simulink model "mech_robot_vr"  (Simulink 7.1)
settings: Solver=ode15s  StartTime=0.0  StopTime=1  RelTol=1e-3  AbsTol=1e-4
PreLoadFcn:
  | load mech_robot_images;mech_robot_data;
undefined symbols (not defined in the file or in its folder): Actuator, rad, s
libraries: mblibv1 x88
(part 3 of 4)

== system mech_robot_vr/Robot/Link 2/Drive2/Continuous angle ==
  Continuous Angle : Subsystem  Tag=Factory continuousAngle  Orientation=left  AncestorBlock=mblibv1/Utilities/Continuous Angle  mask{rad=rad, rads=rad/s}
      mask prompts: rad "Angle measured in:"; rads "Rate measured in:"
      mask help: Outputs a continuous, unbounded angle given a discontinuous, bounded angle and the angular velocity. Choose units for the angle and the angular velocity (rate).
      mask Help: web(mech_help('continuousangle'))
      mask StyleString: popup(rad|deg),popup(rad/s|deg/s)
  Demux : Demux  Orientation=left  Outputs=2
  Joint Sensor : mblibv1/Sensors &  Actuators/Joint Sensor  Orientation=left  DialogController=MECH.DynMechDlgSource  SystemSampleTime=-1  PhysicalDomain=Mechanical  PortType=blob  Muxed=on  Pose=off  Angle=on  AngleUnits=rad  ArcVelocity=on  ArcVelocityUnits=rad/s  ArcAcceleration=off  ArcAccelerationUnits=deg/s^2  CoordPosition=on  CoordPositionUnits=m  Velocity=off  VelocityUnits=m/s  Acceleration=off  AccelerationUnits=m/s^2  Quaternion=on  QuaternionDT=off  QuaternionDDT=off  QuaternionUnits=off  OutputVector=[ 1 1 ]  ActiveIO=on  Width=2  DialogClass=MechanicalSensorBlock  Primitive=R1  Force=off  ForceUnits=N  Torque=off  TorqueUnits=N-m  ReferenceFrame=Absolute (INERTIAL)  ReactionSensedSide=Base  ReactionReferenceFrame=Absolute (World)  ReactionForce=off  ReactionForceUnits=N  ReactionMoment=off  ReactionMomentUnits=N-m
  Mux : Mux  Orientation=left  Inputs=2
  In : PMIOPort  Orientation=left  Port=1  Side=Left
  Out : Outport  Orientation=left  OutDataType=sfix(16)  OutScaling=2^0
  phi : Outport  Orientation=left  Port=2  OutDataType=sfix(16)  OutScaling=2^0
  wires:
  Mux/1 -> Out/1
  Continuous Angle/1(Continuous Angle) -> Mux/1, phi/1
  Demux/2 -> Mux/2, Continuous Angle/2(Rate)
  Demux/1 -> Continuous Angle/1(Angle)
  Joint Sensor/1 -> Demux/1
  connections:
  In/RConn1 -- Joint Sensor/LConn1

== system mech_robot_vr/Robot/Link 2/Drive2/Continuous angle  ==
  Continuous Angle : mblibv1/Utilities/Continuous Angle  Tag=Factory continuousAngle  Orientation=left  SystemSampleTime=-1  rad=rad  rads=rad/s
  Demux : Demux  Orientation=left  Outputs=2
  Gain2 : Gain  Orientation=left  Gain=Actuator.GearRatio  ParameterDataType=sfix(16)  ParameterScaling=2^0  OutDataType=sfix(16)  OutScaling=2^0  SaturateOnIntegerOverflow=on  OutDataTypeStr=Inherit: Same as input  ParamDataTypeStr=Inherit: Same as input
  Joint Sensor : mblibv1/Sensors &  Actuators/Joint Sensor  Orientation=left  DialogController=MECH.DynMechDlgSource  SystemSampleTime=-1  PhysicalDomain=Mechanical  PortType=blob  Muxed=on  Pose=off  Angle=on  AngleUnits=rad  ArcVelocity=on  ArcVelocityUnits=rad/s  ArcAcceleration=off  ArcAccelerationUnits=deg/s^2  CoordPosition=on  CoordPositionUnits=m  Velocity=off  VelocityUnits=m/s  Acceleration=off  AccelerationUnits=m/s^2  Quaternion=on  QuaternionDT=off  QuaternionDDT=off  QuaternionUnits=off  OutputVector=[ 1 1 ]  ActiveIO=on  Width=2  DialogClass=MechanicalSensorBlock  Primitive=R1  Force=off  ForceUnits=N  Torque=off  TorqueUnits=N-m  ReferenceFrame=Absolute (INERTIAL)  ReactionSensedSide=Base  ReactionReferenceFrame=Absolute (World)  ReactionForce=off  ReactionForceUnits=N  ReactionMoment=off  ReactionMomentUnits=N-m
  Mux : Mux  Orientation=left  Inputs=2
  To Workspace : ToWorkspace  VariableName=Body2_D  SampleTime=-1  SaveFormat=Structure With Time
  In : PMIOPort  Orientation=left  Port=1  Side=Left
  "Out " : Outport  Orientation=left  OutDataType=sfix(16)  OutScaling=2^0
  tag scope: Body2=global
  wires:
  Joint Sensor/1 -> Demux/1
  Demux/1 -> Continuous Angle/1
  Demux/2 -> Continuous Angle/2, Mux/2
  Continuous Angle/1 -> Mux/1, [Body2], To Workspace/1
  Mux/1 -> Gain2/1
  Gain2/1 -> "Out "/1
  connections:
  In/RConn1 -- Joint Sensor/LConn1

== system mech_robot_vr/Robot/Link 2/Drive2/Controller ==
  Angular velocity : Inport  OutDataType=sfix(16)  OutScaling=2^0
  w_ref : Inport  Orientation=down  Port=2  OutDataType=sfix(16)  OutScaling=2^0
  phi_ref : Inport  Port=3  OutDataType=sfix(16)  OutScaling=2^0
  phi : Inport  Port=4  OutDataType=sfix(16)  OutScaling=2^0
  Integrator : Integrator  ZeroCross=off
  Lead filter : TransferFcn  Numerator=[340.8*9.95e-3 340.8]  Denominator=[0.56e-3 1]
  Position gain : Gain  Gain=0.3  ParameterDataType=sfix(16)  ParameterScaling=2^0  OutDataType=sfix(16)  OutScaling=2^0  SaturateOnIntegerOverflow=on  OutDataTypeStr=Inherit: Same as input  ParamDataTypeStr=Inherit: Same as input
  Rate controller : TransferFcn  Orientation=up  Numerator=[40e-3 1]  Denominator=[20.2e-3 1]
  Sum : Sum  Inputs=|+-  OutDataType=sfix(16)  OutScaling=2^0  SaturateOnIntegerOverflow=on
  Sum1 : Sum  Inputs=++|  OutDataType=sfix(16)  OutScaling=2^0  SaturateOnIntegerOverflow=on
  Sum2 : Sum  Inputs=|+-  OutDataType=sfix(16)  OutScaling=2^0  SaturateOnIntegerOverflow=on
  Tacho filter : TransferFcn  Numerator=0.03  Denominator="[8.475e-4  1]"
  Taco dynamics : TransferFcn  Numerator=1  Denominator="[1/(2014*2014)   2*0.294/2014  1]"
  Velocity gain : Gain  Orientation=down  Gain=0.03  ParameterDataType=sfix(16)  ParameterScaling=2^0  OutDataType=sfix(16)  OutScaling=2^0  SaturateOnIntegerOverflow=on  OutDataTypeStr=Inherit: Same as input  ParamDataTypeStr=Inherit: Same as input
  i_ref : Outport  OutDataType=sfix(16)  OutScaling=2^0
  wires:
  phi_ref/1 -> Sum/1
  Sum/1 -> Position gain/1
  Position gain/1 -> Sum1/2
  Velocity gain/1 -> Sum1/1
  Sum1/1 -> Sum2/1
  Sum2/1 -> Lead filter/1
  Rate controller/1 -> Sum2/2
  Taco dynamics/1 -> Rate controller/1
  Tacho filter/1 -> Taco dynamics/1
  Angular velocity/1 -> Tacho filter/1
  Lead filter/1 -> Integrator/1
  Integrator/1 -> i_ref/1
  w_ref/1 -> Velocity gain/1
  phi/1 -> Sum/2

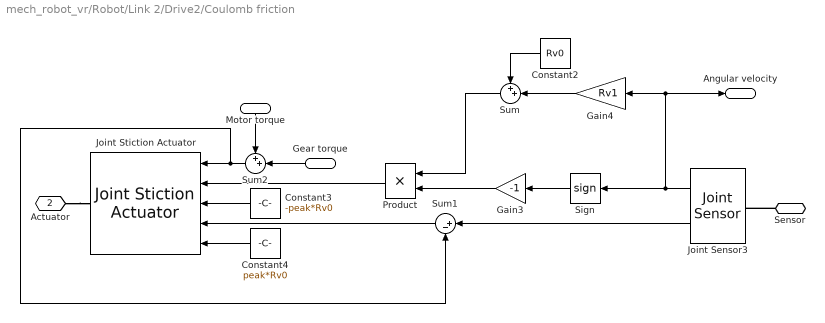
== system mech_robot_vr/Robot/Link 2/Drive2/Coulomb friction ==
  Motor torque : Inport  Orientation=down  OutDataType=sfix(16)  OutScaling=2^0
  Gear torque : Inport  Orientation=left  Port=2  OutDataType=sfix(16)  OutScaling=2^0
  Constant2 : Constant  Orientation=left  Value=Rv0  OutDataType=sfix(16)  OutScaling=2^0
  Constant3 : Constant  Orientation=left  Value=-peak*Rv0  OutDataType=sfix(16)  OutScaling=2^0
  Constant4 : Constant  Orientation=left  Value=peak*Rv0  OutDataType=sfix(16)  OutScaling=2^0
  Gain3 : Gain  Orientation=left  Gain=-1  ParameterDataType=sfix(16)  ParameterScaling=2^0  OutDataType=sfix(16)  OutScaling=2^0  SaturateOnIntegerOverflow=on  OutDataTypeStr=Inherit: Same as input  ParamDataTypeStr=Inherit: Same as input
  Gain4 : Gain  Orientation=left  Gain=Rv1  ParameterDataType=sfix(16)  ParameterScaling=2^0  OutDataType=sfix(16)  OutScaling=2^0  SaturateOnIntegerOverflow=on  OutDataTypeStr=Inherit: Same as input  ParamDataTypeStr=Inherit: Same as input
  Joint Sensor3 : mblibv1/Sensors &  Actuators/Joint Sensor  Description=Mechanical Blockset  Orientation=left  DialogController=MECH.DynMechDlgSource  SystemSampleTime=-1  PhysicalDomain=Mechanical  PortType=blob  Muxed=off  Pose=off  Angle=off  AngleUnits=rad  ArcVelocity=on  ArcVelocityUnits=rad/s  ArcAcceleration=off  ArcAccelerationUnits=deg/s^2  CoordPosition=off  CoordPositionUnits=m  Velocity=off  VelocityUnits=m/s  Acceleration=off  AccelerationUnits=m/s^2  Quaternion=off  QuaternionDT=off  QuaternionDDT=off  QuaternionUnits=off  OutputVector=[ 1 1 ]  ActiveIO=on  Width=2  DialogClass=MechanicalSensorBlock  Primitive=R1  Force=off  ForceUnits=N  Torque=on  TorqueUnits=N-m  ReferenceFrame=Absolute (INERTIAL)  ReactionSensedSide=Base  ReactionReferenceFrame=Absolute (World)  ReactionForce=off  ReactionForceUnits=N  ReactionMoment=off  ReactionMomentUnits=N-m
  Joint Stiction Actuator : mblibv1/Sensors &  Actuators/Joint Stiction Actuator  Description=Mechanical Blockset  Orientation=left  DialogController=MECH.DynMechDlgSource  SystemSampleTime=-1  PhysicalDomain=Mechanical  PortType=blob  ActuationStyle=Force  AngleUnits=deg  ArcVelocityUnits=deg/s  ArcAccelerationUnits=deg/s^2  CoordPositionUnits=m  VelocityUnits=m/s  AccelerationUnits=m/s^2  ForceUnits=N  TorqueUnits=N-m  ActiveIO=on  Width=5  DialogClass=EventActuatorBlock  Primitive=R1  FrictionalForceUnits=N  ExternalForceUnits=N  FrictionalTorqueUnits=N-m  ExternalTorqueUnits=N-m  LockingTolerance=1e-3
  Product : Product  Orientation=left  OutDataType=sfix(16)  OutScaling=2^0  SaturateOnIntegerOverflow=on  InputSameDT=on  OutDataTypeStr=Inherit: Same as first input
  Sign : Signum  Orientation=left
  Sum : Sum  Orientation=left  Inputs=++|  OutDataType=sfix(16)  OutScaling=2^0  SaturateOnIntegerOverflow=on  InputSameDT=on  OutDataTypeStr=Inherit: Same as first input
  Sum1 : Sum  Orientation=left  Inputs=|+-  OutDataType=sfix(16)  OutScaling=2^0  SaturateOnIntegerOverflow=on  InputSameDT=on  OutDataTypeStr=Inherit: Same as first input
  Sum2 : Sum  Orientation=left  Inputs=++|  OutDataType=sfix(16)  OutScaling=2^0  SaturateOnIntegerOverflow=on
  Sensor : PMIOPort  Orientation=left  Port=1  Side=Right
  Actuator : PMIOPort  Port=2  Side=Right
  Angular velocity : Outport  OutDataType=sfix(16)  OutScaling=2^0
  wires:
  Sum1/1 -> Joint Stiction Actuator/4
  Constant3/1 -> Joint Stiction Actuator/3
  Gain3/1 -> Product/2
  Constant2/1 -> Sum/1
  Gain4/1 -> Sum/2
  Constant4/1 -> Joint Stiction Actuator/5
  Joint Sensor3/2 -> Sum1/1
  Sum/1 -> Product/1
  Sign/1 -> Gain3/1
  Product/1 -> Joint Stiction Actuator/2
  Motor torque/1 -> Sum2/1
  Gear torque/1 -> Sum2/2
  Sum2/1 -> Joint Stiction Actuator/1, Sum1/2
  Joint Sensor3/1 -> Sign/1, Gain4/1, Angular velocity/1
  connections:
  Sensor/RConn1 -- Joint Sensor3/LConn1
  Actuator/RConn1 -- Joint Stiction Actuator/RConn1

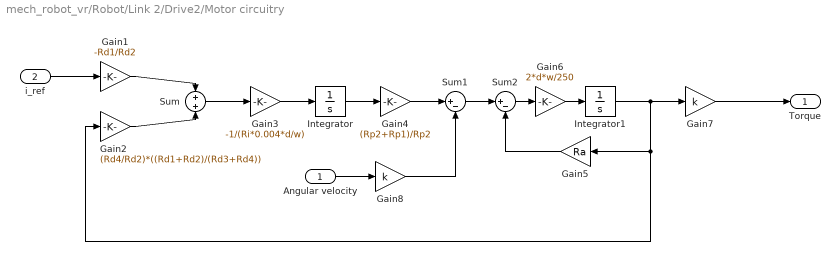
== system mech_robot_vr/Robot/Link 2/Drive2/Motor circuitry ==
  Angular velocity : Inport  OutDataType=sfix(16)  OutScaling=2^0
  i_ref : Inport  Port=2  OutDataType=sfix(16)  OutScaling=2^0
  Gain1 : Gain  Gain=-Rd1/Rd2  ParameterDataType=sfix(16)  ParameterScaling=2^0  OutDataType=sfix(16)  OutScaling=2^0  SaturateOnIntegerOverflow=on  OutDataTypeStr=Inherit: Same as input  ParamDataTypeStr=Inherit: Same as input
  Gain2 : Gain  Gain=(Rd4/Rd2)*((Rd1+Rd2)/(Rd3+Rd4))  ParameterDataType=sfix(16)  ParameterScaling=2^0  OutDataType=sfix(16)  OutScaling=2^0  SaturateOnIntegerOverflow=on  OutDataTypeStr=Inherit: Same as input  ParamDataTypeStr=Inherit: Same as input
  Gain3 : Gain  Gain=-1/(Ri*0.004*d/w)  ParameterDataType=sfix(16)  ParameterScaling=2^0  OutDataType=sfix(16)  OutScaling=2^0  SaturateOnIntegerOverflow=on  OutDataTypeStr=Inherit: Same as input  ParamDataTypeStr=Inherit: Same as input
  Gain4 : Gain  Gain=(Rp2+Rp1)/Rp2  ParameterDataType=sfix(16)  ParameterScaling=2^0  OutDataType=sfix(16)  OutScaling=2^0  SaturateOnIntegerOverflow=on  OutDataTypeStr=Inherit: Same as input  ParamDataTypeStr=Inherit: Same as input
  Gain5 : Gain  Orientation=left  Gain=Ra  ParameterDataType=sfix(16)  ParameterScaling=2^0  OutDataType=sfix(16)  OutScaling=2^0  SaturateOnIntegerOverflow=on  OutDataTypeStr=Inherit: Same as input  ParamDataTypeStr=Inherit: Same as input
  Gain6 : Gain  Gain=2*d*w/250  ParameterDataType=sfix(16)  ParameterScaling=2^0  OutDataType=sfix(16)  OutScaling=2^0  SaturateOnIntegerOverflow=on  OutDataTypeStr=Inherit: Same as input  ParamDataTypeStr=Inherit: Same as input
  Gain7 : Gain  Gain=k  ParameterDataType=sfix(16)  ParameterScaling=2^0  OutDataType=sfix(16)  OutScaling=2^0  SaturateOnIntegerOverflow=on  OutDataTypeStr=Inherit: Same as input  ParamDataTypeStr=Inherit: Same as input
  Gain8 : Gain  Gain=k  ParameterDataType=sfix(16)  ParameterScaling=2^0  OutDataType=sfix(16)  OutScaling=2^0  SaturateOnIntegerOverflow=on  OutDataTypeStr=Inherit: Same as input  ParamDataTypeStr=Inherit: Same as input
  Integrator : Integrator  ZeroCross=off
  Integrator1 : Integrator  ZeroCross=off
  Sum : Sum  OutDataType=sfix(16)  OutScaling=2^0  SaturateOnIntegerOverflow=on  InputSameDT=on  OutDataTypeStr=Inherit: Same as first input
  Sum1 : Sum  Inputs=|+-  OutDataType=sfix(16)  OutScaling=2^0  SaturateOnIntegerOverflow=on  InputSameDT=on  OutDataTypeStr=Inherit: Same as first input
  Sum2 : Sum  Inputs=|+-  OutDataType=sfix(16)  OutScaling=2^0  SaturateOnIntegerOverflow=on  InputSameDT=on  OutDataTypeStr=Inherit: Same as first input
  Torque : Outport  OutDataType=sfix(16)  OutScaling=2^0
  wires:
  Angular velocity/1 -> Gain8/1
  Gain8/1 -> Sum1/2
  Gain6/1 -> Integrator1/1
  Sum2/1 -> Gain6/1
  Gain5/1 -> Sum2/2
  Integrator1/1 -> Gain2/1, Gain5/1, Gain7/1
  Sum1/1 -> Sum2/1
  Gain4/1 -> Sum1/1
  Integrator/1 -> Gain4/1
  Gain3/1 -> Integrator/1
  Sum/1 -> Gain3/1
  Gain2/1 -> Sum/2
  Gain1/1 -> Sum/1
  i_ref/1 -> Gain1/1
  Gain7/1 -> Torque/1

== system mech_robot_vr/Robot/Link3/Drive3/Continuous angle ==
  Continuous Angle : Subsystem  Tag=Factory continuousAngle  Orientation=left  AncestorBlock=mblibv1/Utilities/Continuous Angle  mask{rad=rad, rads=rad/s}
      mask prompts: rad "Angle measured in:"; rads "Rate measured in:"
      mask help: Outputs a continuous, unbounded angle given a discontinuous, bounded angle and the angular velocity. Choose units for the angle and the angular velocity (rate).
      mask Help: web(mech_help('continuousangle'))
      mask StyleString: popup(rad|deg),popup(rad/s|deg/s)
  Demux : Demux  Orientation=left  Outputs=2
  Joint Sensor : mblibv1/Sensors &  Actuators/Joint Sensor  Orientation=left  DialogController=MECH.DynMechDlgSource  SystemSampleTime=-1  PhysicalDomain=Mechanical  PortType=blob  Muxed=on  Pose=off  Angle=on  AngleUnits=rad  ArcVelocity=on  ArcVelocityUnits=rad/s  ArcAcceleration=off  ArcAccelerationUnits=deg/s^2  CoordPosition=on  CoordPositionUnits=m  Velocity=off  VelocityUnits=m/s  Acceleration=off  AccelerationUnits=m/s^2  Quaternion=on  QuaternionDT=off  QuaternionDDT=off  QuaternionUnits=off  OutputVector=[ 1 1 ]  ActiveIO=on  Width=2  DialogClass=MechanicalSensorBlock  Primitive=R1  Force=off  ForceUnits=N  Torque=off  TorqueUnits=N-m  ReferenceFrame=Absolute (INERTIAL)  ReactionSensedSide=Base  ReactionReferenceFrame=Absolute (World)  ReactionForce=off  ReactionForceUnits=N  ReactionMoment=off  ReactionMomentUnits=N-m
  Mux : Mux  Orientation=left  Inputs=2
  In : PMIOPort  Orientation=left  Port=1  Side=Left
  Out : Outport  Orientation=left  OutDataType=sfix(16)  OutScaling=2^0
  phi : Outport  Orientation=left  Port=2  OutDataType=sfix(16)  OutScaling=2^0
  wires:
  Mux/1 -> Out/1
  Continuous Angle/1(Continuous Angle) -> Mux/1, phi/1
  Demux/2 -> Mux/2, Continuous Angle/2(Rate)
  Demux/1 -> Continuous Angle/1(Angle)
  Joint Sensor/1 -> Demux/1
  connections:
  In/RConn1 -- Joint Sensor/LConn1

== system mech_robot_vr/Robot/Link3/Drive3/Continuous angle  ==
  Continuous Angle : mblibv1/Utilities/Continuous Angle  Tag=Factory continuousAngle  Orientation=left  SystemSampleTime=-1  rad=rad  rads=rad/s
  Demux : Demux  Orientation=left  Outputs=2
  Gain2 : Gain  Orientation=left  Gain=Actuator.GearRatio  ParameterDataType=sfix(16)  ParameterScaling=2^0  OutDataType=sfix(16)  OutScaling=2^0  SaturateOnIntegerOverflow=on  OutDataTypeStr=Inherit: Same as input  ParamDataTypeStr=Inherit: Same as input
  Joint Sensor : mblibv1/Sensors &  Actuators/Joint Sensor  Orientation=left  DialogController=MECH.DynMechDlgSource  SystemSampleTime=-1  PhysicalDomain=Mechanical  PortType=blob  Muxed=on  Pose=off  Angle=on  AngleUnits=rad  ArcVelocity=on  ArcVelocityUnits=rad/s  ArcAcceleration=off  ArcAccelerationUnits=deg/s^2  CoordPosition=on  CoordPositionUnits=m  Velocity=off  VelocityUnits=m/s  Acceleration=off  AccelerationUnits=m/s^2  Quaternion=on  QuaternionDT=off  QuaternionDDT=off  QuaternionUnits=off  OutputVector=[ 1 1 ]  ActiveIO=on  Width=2  DialogClass=MechanicalSensorBlock  Primitive=R1  Force=off  ForceUnits=N  Torque=off  TorqueUnits=N-m  ReferenceFrame=Absolute (INERTIAL)  ReactionSensedSide=Base  ReactionReferenceFrame=Absolute (World)  ReactionForce=off  ReactionForceUnits=N  ReactionMoment=off  ReactionMomentUnits=N-m
  Mux : Mux  Orientation=left  Inputs=2
  To Workspace : ToWorkspace  VariableName=Body3_D  SampleTime=-1  SaveFormat=Structure With Time
  In : PMIOPort  Orientation=left  Port=1  Side=Left
  "Out " : Outport  Orientation=left  OutDataType=sfix(16)  OutScaling=2^0
  tag scope: Body3=global
  wires:
  Joint Sensor/1 -> Demux/1
  Demux/1 -> Continuous Angle/1
  Demux/2 -> Continuous Angle/2, Mux/2
  Continuous Angle/1 -> Mux/1, [Body3], To Workspace/1
  Mux/1 -> Gain2/1
  Gain2/1 -> "Out "/1
  connections:
  In/RConn1 -- Joint Sensor/LConn1

== system mech_robot_vr/Robot/Link3/Drive3/Controller ==
  Angular velocity : Inport  OutDataType=sfix(16)  OutScaling=2^0
  w_ref : Inport  Orientation=down  Port=2  OutDataType=sfix(16)  OutScaling=2^0
  phi_ref : Inport  Port=3  OutDataType=sfix(16)  OutScaling=2^0
  phi : Inport  Port=4  OutDataType=sfix(16)  OutScaling=2^0
  Integrator : Integrator  ZeroCross=off
  Lead filter : TransferFcn  Numerator=[340.8*9.95e-3 340.8]  Denominator=[0.56e-3 1]
  Position gain : Gain  Gain=0.3  ParameterDataType=sfix(16)  ParameterScaling=2^0  OutDataType=sfix(16)  OutScaling=2^0  SaturateOnIntegerOverflow=on  OutDataTypeStr=Inherit: Same as input  ParamDataTypeStr=Inherit: Same as input
  Rate controller : TransferFcn  Orientation=up  Numerator=[40e-3 1]  Denominator=[20.2e-3 1]
  Sum : Sum  Inputs=|+-  OutDataType=sfix(16)  OutScaling=2^0  SaturateOnIntegerOverflow=on
  Sum1 : Sum  Inputs=++|  OutDataType=sfix(16)  OutScaling=2^0  SaturateOnIntegerOverflow=on
  Sum2 : Sum  Inputs=|+-  OutDataType=sfix(16)  OutScaling=2^0  SaturateOnIntegerOverflow=on
  Tacho filter : TransferFcn  Numerator=0.03  Denominator="[8.475e-4  1]"
  Taco dynamics : TransferFcn  Numerator=1  Denominator="[1/(2014*2014)   2*0.294/2014  1]"
  Velocity gain : Gain  Orientation=down  Gain=0.03  ParameterDataType=sfix(16)  ParameterScaling=2^0  OutDataType=sfix(16)  OutScaling=2^0  SaturateOnIntegerOverflow=on  OutDataTypeStr=Inherit: Same as input  ParamDataTypeStr=Inherit: Same as input
  i_ref : Outport  OutDataType=sfix(16)  OutScaling=2^0
  wires:
  phi_ref/1 -> Sum/1
  Sum/1 -> Position gain/1
  Position gain/1 -> Sum1/2
  Velocity gain/1 -> Sum1/1
  Sum1/1 -> Sum2/1
  Sum2/1 -> Lead filter/1
  Rate controller/1 -> Sum2/2
  Taco dynamics/1 -> Rate controller/1
  Tacho filter/1 -> Taco dynamics/1
  Angular velocity/1 -> Tacho filter/1
  Lead filter/1 -> Integrator/1
  Integrator/1 -> i_ref/1
  w_ref/1 -> Velocity gain/1
  phi/1 -> Sum/2

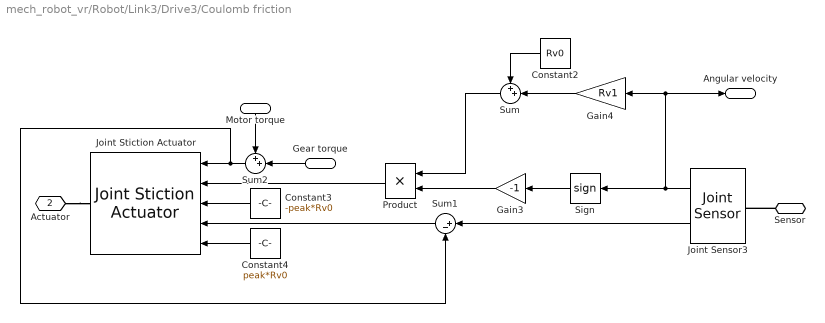
== system mech_robot_vr/Robot/Link3/Drive3/Coulomb friction ==
  Motor torque : Inport  Orientation=down  OutDataType=sfix(16)  OutScaling=2^0
  Gear torque : Inport  Orientation=left  Port=2  OutDataType=sfix(16)  OutScaling=2^0
  Constant2 : Constant  Orientation=left  Value=Rv0  OutDataType=sfix(16)  OutScaling=2^0
  Constant3 : Constant  Orientation=left  Value=-peak*Rv0  OutDataType=sfix(16)  OutScaling=2^0
  Constant4 : Constant  Orientation=left  Value=peak*Rv0  OutDataType=sfix(16)  OutScaling=2^0
  Gain3 : Gain  Orientation=left  Gain=-1  ParameterDataType=sfix(16)  ParameterScaling=2^0  OutDataType=sfix(16)  OutScaling=2^0  SaturateOnIntegerOverflow=on  OutDataTypeStr=Inherit: Same as input  ParamDataTypeStr=Inherit: Same as input
  Gain4 : Gain  Orientation=left  Gain=Rv1  ParameterDataType=sfix(16)  ParameterScaling=2^0  OutDataType=sfix(16)  OutScaling=2^0  SaturateOnIntegerOverflow=on  OutDataTypeStr=Inherit: Same as input  ParamDataTypeStr=Inherit: Same as input
  Joint Sensor3 : mblibv1/Sensors &  Actuators/Joint Sensor  Description=Mechanical Blockset  Orientation=left  DialogController=MECH.DynMechDlgSource  SystemSampleTime=-1  PhysicalDomain=Mechanical  PortType=blob  Muxed=off  Pose=off  Angle=off  AngleUnits=rad  ArcVelocity=on  ArcVelocityUnits=rad/s  ArcAcceleration=off  ArcAccelerationUnits=deg/s^2  CoordPosition=off  CoordPositionUnits=m  Velocity=off  VelocityUnits=m/s  Acceleration=off  AccelerationUnits=m/s^2  Quaternion=off  QuaternionDT=off  QuaternionDDT=off  QuaternionUnits=off  OutputVector=[ 1 1 ]  ActiveIO=on  Width=2  DialogClass=MechanicalSensorBlock  Primitive=R1  Force=off  ForceUnits=N  Torque=on  TorqueUnits=N-m  ReferenceFrame=Absolute (INERTIAL)  ReactionSensedSide=Base  ReactionReferenceFrame=Absolute (World)  ReactionForce=off  ReactionForceUnits=N  ReactionMoment=off  ReactionMomentUnits=N-m
  Joint Stiction Actuator : mblibv1/Sensors &  Actuators/Joint Stiction Actuator  Description=Mechanical Blockset  Orientation=left  DialogController=MECH.DynMechDlgSource  SystemSampleTime=-1  PhysicalDomain=Mechanical  PortType=blob  ActuationStyle=Force  AngleUnits=deg  ArcVelocityUnits=deg/s  ArcAccelerationUnits=deg/s^2  CoordPositionUnits=m  VelocityUnits=m/s  AccelerationUnits=m/s^2  ForceUnits=N  TorqueUnits=N-m  ActiveIO=on  Width=5  DialogClass=EventActuatorBlock  Primitive=R1  FrictionalForceUnits=N  ExternalForceUnits=N  FrictionalTorqueUnits=N-m  ExternalTorqueUnits=N-m  LockingTolerance=1e-3
  Product : Product  Orientation=left  OutDataType=sfix(16)  OutScaling=2^0  SaturateOnIntegerOverflow=on  InputSameDT=on  OutDataTypeStr=Inherit: Same as first input
  Sign : Signum  Orientation=left
  Sum : Sum  Orientation=left  Inputs=++|  OutDataType=sfix(16)  OutScaling=2^0  SaturateOnIntegerOverflow=on  InputSameDT=on  OutDataTypeStr=Inherit: Same as first input
  Sum1 : Sum  Orientation=left  Inputs=|+-  OutDataType=sfix(16)  OutScaling=2^0  SaturateOnIntegerOverflow=on  InputSameDT=on  OutDataTypeStr=Inherit: Same as first input
  Sum2 : Sum  Orientation=left  Inputs=++|  OutDataType=sfix(16)  OutScaling=2^0  SaturateOnIntegerOverflow=on
  Sensor : PMIOPort  Orientation=left  Port=1  Side=Right
  Actuator : PMIOPort  Port=2  Side=Right
  Angular velocity : Outport  OutDataType=sfix(16)  OutScaling=2^0
  wires:
  Sum1/1 -> Joint Stiction Actuator/4
  Constant3/1 -> Joint Stiction Actuator/3
  Gain3/1 -> Product/2
  Constant2/1 -> Sum/1
  Gain4/1 -> Sum/2
  Constant4/1 -> Joint Stiction Actuator/5
  Joint Sensor3/2 -> Sum1/1
  Sum/1 -> Product/1
  Sign/1 -> Gain3/1
  Product/1 -> Joint Stiction Actuator/2
  Motor torque/1 -> Sum2/1
  Gear torque/1 -> Sum2/2
  Sum2/1 -> Joint Stiction Actuator/1, Sum1/2
  Joint Sensor3/1 -> Sign/1, Gain4/1, Angular velocity/1
  connections:
  Sensor/RConn1 -- Joint Sensor3/LConn1
  Actuator/RConn1 -- Joint Stiction Actuator/RConn1

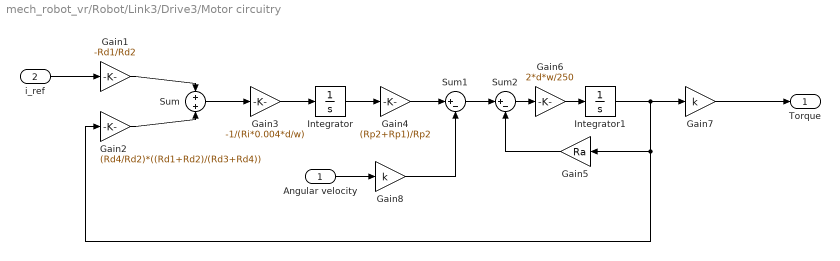
== system mech_robot_vr/Robot/Link3/Drive3/Motor circuitry ==
  Angular velocity : Inport  OutDataType=sfix(16)  OutScaling=2^0
  i_ref : Inport  Port=2  OutDataType=sfix(16)  OutScaling=2^0
  Gain1 : Gain  Gain=-Rd1/Rd2  ParameterDataType=sfix(16)  ParameterScaling=2^0  OutDataType=sfix(16)  OutScaling=2^0  SaturateOnIntegerOverflow=on  OutDataTypeStr=Inherit: Same as input  ParamDataTypeStr=Inherit: Same as input
  Gain2 : Gain  Gain=(Rd4/Rd2)*((Rd1+Rd2)/(Rd3+Rd4))  ParameterDataType=sfix(16)  ParameterScaling=2^0  OutDataType=sfix(16)  OutScaling=2^0  SaturateOnIntegerOverflow=on  OutDataTypeStr=Inherit: Same as input  ParamDataTypeStr=Inherit: Same as input
  Gain3 : Gain  Gain=-1/(Ri*0.004*d/w)  ParameterDataType=sfix(16)  ParameterScaling=2^0  OutDataType=sfix(16)  OutScaling=2^0  SaturateOnIntegerOverflow=on  OutDataTypeStr=Inherit: Same as input  ParamDataTypeStr=Inherit: Same as input
  Gain4 : Gain  Gain=(Rp2+Rp1)/Rp2  ParameterDataType=sfix(16)  ParameterScaling=2^0  OutDataType=sfix(16)  OutScaling=2^0  SaturateOnIntegerOverflow=on  OutDataTypeStr=Inherit: Same as input  ParamDataTypeStr=Inherit: Same as input
  Gain5 : Gain  Orientation=left  Gain=Ra  ParameterDataType=sfix(16)  ParameterScaling=2^0  OutDataType=sfix(16)  OutScaling=2^0  SaturateOnIntegerOverflow=on  OutDataTypeStr=Inherit: Same as input  ParamDataTypeStr=Inherit: Same as input
  Gain6 : Gain  Gain=2*d*w/250  ParameterDataType=sfix(16)  ParameterScaling=2^0  OutDataType=sfix(16)  OutScaling=2^0  SaturateOnIntegerOverflow=on  OutDataTypeStr=Inherit: Same as input  ParamDataTypeStr=Inherit: Same as input
  Gain7 : Gain  Gain=k  ParameterDataType=sfix(16)  ParameterScaling=2^0  OutDataType=sfix(16)  OutScaling=2^0  SaturateOnIntegerOverflow=on  OutDataTypeStr=Inherit: Same as input  ParamDataTypeStr=Inherit: Same as input
  Gain8 : Gain  Gain=k  ParameterDataType=sfix(16)  ParameterScaling=2^0  OutDataType=sfix(16)  OutScaling=2^0  SaturateOnIntegerOverflow=on  OutDataTypeStr=Inherit: Same as input  ParamDataTypeStr=Inherit: Same as input
  Integrator : Integrator  ZeroCross=off
  Integrator1 : Integrator  ZeroCross=off
  Sum : Sum  OutDataType=sfix(16)  OutScaling=2^0  SaturateOnIntegerOverflow=on  InputSameDT=on  OutDataTypeStr=Inherit: Same as first input
  Sum1 : Sum  Inputs=|+-  OutDataType=sfix(16)  OutScaling=2^0  SaturateOnIntegerOverflow=on  InputSameDT=on  OutDataTypeStr=Inherit: Same as first input
  Sum2 : Sum  Inputs=|+-  OutDataType=sfix(16)  OutScaling=2^0  SaturateOnIntegerOverflow=on  InputSameDT=on  OutDataTypeStr=Inherit: Same as first input
  Torque : Outport  OutDataType=sfix(16)  OutScaling=2^0
  wires:
  Angular velocity/1 -> Gain8/1
  Gain8/1 -> Sum1/2
  Gain6/1 -> Integrator1/1
  Sum2/1 -> Gain6/1
  Gain5/1 -> Sum2/2
  Integrator1/1 -> Gain2/1, Gain5/1, Gain7/1
  Sum1/1 -> Sum2/1
  Gain4/1 -> Sum1/1
  Integrator/1 -> Gain4/1
  Gain3/1 -> Integrator/1
  Sum/1 -> Gain3/1
  Gain2/1 -> Sum/2
  Gain1/1 -> Sum/1
  i_ref/1 -> Gain1/1
  Gain7/1 -> Torque/1

== system mech_robot_vr/Robot/Link4/Drive4/Continuous angle ==
  Angular velocity : Inport  Orientation=left  OutDataType=sfix(16)  OutScaling=2^0
  phi : Inport  Orientation=left  Port=2  OutDataType=sfix(16)  OutScaling=2^0
  Continuous Angle : Subsystem  Tag=Factory continuousAngle  Orientation=left  AncestorBlock=mblibv1/Utilities/Continuous Angle  mask{rad=rad, rads=rad/s}
      mask prompts: rad "Angle measured in:"; rads "Rate measured in:"
      mask help: Outputs a continuous, unbounded angle given a discontinuous, bounded angle and the angular velocity. Choose units for the angle and the angular velocity (rate).
      mask Help: web(mech_help('continuousangle'))
      mask StyleString: popup(rad|deg),popup(rad/s|deg/s)
  "phi " : Outport  Orientation=left  OutDataType=sfix(16)  OutScaling=2^0
  "Angular velocity " : Outport  Orientation=left  Port=2  OutDataType=sfix(16)  OutScaling=2^0
  wires:
  Continuous Angle/1(Continuous Angle) -> "phi "/1
  phi/1 -> Continuous Angle/1(Angle)
  Angular velocity/1 -> Continuous Angle/2(Rate), "Angular velocity "/1

== system mech_robot_vr/Robot/Link4/Drive4/Controller ==
  Angular velocity : Inport  OutDataType=sfix(16)  OutScaling=2^0
  phi : Inport  Port=2  OutDataType=sfix(16)  OutScaling=2^0
  w_ref : Inport  Orientation=down  Port=3  OutDataType=sfix(16)  OutScaling=2^0
  phi_ref : Inport  Port=4  OutDataType=sfix(16)  OutScaling=2^0
  Integrator : Integrator  ZeroCross=off
  Lead filter : TransferFcn  Numerator=[340.8*9.95e-3 340.8]  Denominator=[0.56e-3 1]
  Position gain : Gain  Gain=0.3  ParameterDataType=sfix(16)  ParameterScaling=2^0  OutDataType=sfix(16)  OutScaling=2^0  SaturateOnIntegerOverflow=on  OutDataTypeStr=Inherit: Same as input  ParamDataTypeStr=Inherit: Same as input
  Rate controller : TransferFcn  Orientation=up  Numerator=[40e-3 1]  Denominator=[20.2e-3 1]
  Sum : Sum  Inputs=|+-  OutDataType=sfix(16)  OutScaling=2^0  SaturateOnIntegerOverflow=on
  Sum1 : Sum  Inputs=++|  OutDataType=sfix(16)  OutScaling=2^0  SaturateOnIntegerOverflow=on
  Sum2 : Sum  Inputs=|+-  OutDataType=sfix(16)  OutScaling=2^0  SaturateOnIntegerOverflow=on
  Tacho filter : TransferFcn  Numerator=0.03  Denominator="[8.475e-4  1]"
  Taco dynamics : TransferFcn  Numerator=1  Denominator="[1/(2014*2014)   2*0.294/2014  1]"
  Velocity gain : Gain  Orientation=down  Gain=0.03  ParameterDataType=sfix(16)  ParameterScaling=2^0  OutDataType=sfix(16)  OutScaling=2^0  SaturateOnIntegerOverflow=on  OutDataTypeStr=Inherit: Same as input  ParamDataTypeStr=Inherit: Same as input
  i_ref : Outport  OutDataType=sfix(16)  OutScaling=2^0
  wires:
  phi_ref/1 -> Sum/1
  Sum/1 -> Position gain/1
  Position gain/1 -> Sum1/2
  Velocity gain/1 -> Sum1/1
  Sum1/1 -> Sum2/1
  Sum2/1 -> Lead filter/1
  Rate controller/1 -> Sum2/2
  Taco dynamics/1 -> Rate controller/1
  Tacho filter/1 -> Taco dynamics/1
  Angular velocity/1 -> Tacho filter/1
  Lead filter/1 -> Integrator/1
  Integrator/1 -> i_ref/1
  w_ref/1 -> Velocity gain/1
  phi/1 -> Sum/2

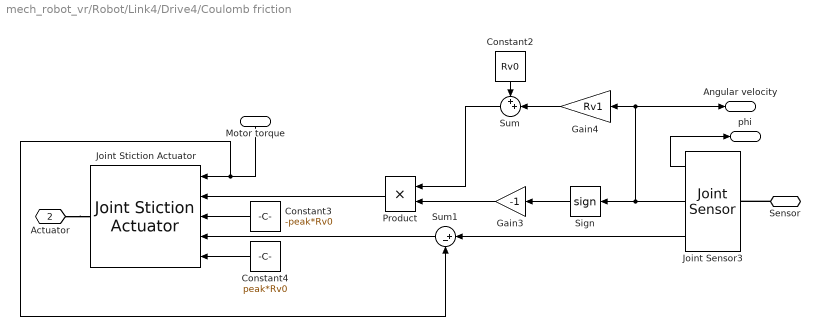
== system mech_robot_vr/Robot/Link4/Drive4/Coulomb friction ==
  Motor torque : Inport  Orientation=down  OutDataType=sfix(16)  OutScaling=2^0
  Constant2 : Constant  Orientation=down  Value=Rv0  OutDataType=sfix(16)  OutScaling=2^0
  Constant3 : Constant  Orientation=left  Value=-peak*Rv0  OutDataType=sfix(16)  OutScaling=2^0
  Constant4 : Constant  Orientation=left  Value=peak*Rv0  OutDataType=sfix(16)  OutScaling=2^0
  Gain3 : Gain  Orientation=left  Gain=-1  ParameterDataType=sfix(16)  ParameterScaling=2^0  OutDataType=sfix(16)  OutScaling=2^0  SaturateOnIntegerOverflow=on  OutDataTypeStr=Inherit: Same as input  ParamDataTypeStr=Inherit: Same as input
  Gain4 : Gain  Orientation=left  Gain=Rv1  ParameterDataType=sfix(16)  ParameterScaling=2^0  OutDataType=sfix(16)  OutScaling=2^0  SaturateOnIntegerOverflow=on  OutDataTypeStr=Inherit: Same as input  ParamDataTypeStr=Inherit: Same as input
  Joint Sensor3 : mblibv1/Sensors &  Actuators/Joint Sensor  Description=Mechanical Blockset  Orientation=left  DialogController=MECH.DynMechDlgSource  SystemSampleTime=-1  PhysicalDomain=Mechanical  PortType=blob  Muxed=off  Pose=off  Angle=on  AngleUnits=rad  ArcVelocity=on  ArcVelocityUnits=rad/s  ArcAcceleration=off  ArcAccelerationUnits=deg/s^2  CoordPosition=off  CoordPositionUnits=m  Velocity=off  VelocityUnits=m/s  Acceleration=off  AccelerationUnits=m/s^2  Quaternion=off  QuaternionDT=off  QuaternionDDT=off  QuaternionUnits=off  OutputVector=[ 1 1 1 ]  ActiveIO=on  Width=3  DialogClass=MechanicalSensorBlock  Primitive=R1  Force=off  ForceUnits=N  Torque=on  TorqueUnits=N-m  ReferenceFrame=Absolute (INERTIAL)  ReactionSensedSide=Base  ReactionReferenceFrame=Absolute (World)  ReactionForce=off  ReactionForceUnits=N  ReactionMoment=off  ReactionMomentUnits=N-m
  Joint Stiction Actuator : mblibv1/Sensors &  Actuators/Joint Stiction Actuator  Description=Mechanical Blockset  Orientation=left  DialogController=MECH.DynMechDlgSource  SystemSampleTime=-1  PhysicalDomain=Mechanical  PortType=blob  ActuationStyle=Force  AngleUnits=deg  ArcVelocityUnits=deg/s  ArcAccelerationUnits=deg/s^2  CoordPositionUnits=m  VelocityUnits=m/s  AccelerationUnits=m/s^2  ForceUnits=N  TorqueUnits=N-m  ActiveIO=on  Width=5  DialogClass=EventActuatorBlock  Primitive=R1  FrictionalForceUnits=N  ExternalForceUnits=N  FrictionalTorqueUnits=N-m  ExternalTorqueUnits=N-m  LockingTolerance=1e-3
  Product : Product  Orientation=left  OutDataType=sfix(16)  OutScaling=2^0  SaturateOnIntegerOverflow=on  InputSameDT=on  OutDataTypeStr=Inherit: Same as first input
  Sign : Signum  Orientation=left
  Sum : Sum  Orientation=left  Inputs=++|  OutDataType=sfix(16)  OutScaling=2^0  SaturateOnIntegerOverflow=on  InputSameDT=on  OutDataTypeStr=Inherit: Same as first input
  Sum1 : Sum  Orientation=left  Inputs=|+-  OutDataType=sfix(16)  OutScaling=2^0  SaturateOnIntegerOverflow=on  InputSameDT=on  OutDataTypeStr=Inherit: Same as first input
  Sensor : PMIOPort  Orientation=left  Port=1  Side=Right
  Actuator : PMIOPort  Port=2  Side=Right
  phi : Outport  OutDataType=sfix(16)  OutScaling=2^0
  Angular velocity : Outport  Port=2  OutDataType=sfix(16)  OutScaling=2^0
  wires:
  Sum1/1 -> Joint Stiction Actuator/4
  Constant3/1 -> Joint Stiction Actuator/3
  Gain3/1 -> Product/2
  Constant2/1 -> Sum/1
  Gain4/1 -> Sum/2
  Constant4/1 -> Joint Stiction Actuator/5
  Sum/1 -> Product/1
  Sign/1 -> Gain3/1
  Product/1 -> Joint Stiction Actuator/2
  Motor torque/1 -> Joint Stiction Actuator/1, Sum1/2
  Joint Sensor3/2 -> Sign/1, Gain4/1, Angular velocity/1
  Joint Sensor3/3 -> Sum1/1
  Joint Sensor3/1 -> phi/1
  connections:
  Sensor/RConn1 -- Joint Sensor3/LConn1
  Actuator/RConn1 -- Joint Stiction Actuator/RConn1

== system mech_robot_vr/Robot/Link4/Drive4/Ideal gear ==
  "Continuous angle " : Subsystem  Orientation=left
  Gear : mblibv1/Bodies/Body  Tag=Factory generic  Description=Mechanical Blockset  Orientation=left  DialogController=MECH.DynMechDlgSource  PhysicalDomain=mechanical  SubClassName=Unknown  LeftPortType=workingframe  RightPortType=workingframe  LConnTagsString=CS1  RConnTagsString=CS2|CS3  DialogClass=MechanicalBodyBlock  Mass=0  MassUnits=kg  InertiaUnits=kg*m^2  Inertia=zeros(3,3)  Shape=Cylinder  ShapeDims=[1 1]  ShapeUnits=m  ShapeUse=false  Density=1  DensityUnits=kg/m^3  DensityUse=false  GraphicsMode=1  BodyColor=[0.5 0.5 0.5]  GraphicsObj=[]  AttachedToCS=1  CG=Left$CG$[0 0 0]$CS1$CS1$m$[0 0 0]$Euler X-Y-Z$deg$WORLD$false  WorkingFrames=Left$CS1$[0 0 0]$ADJOINING$ADJOINING$m$[0 0 0]$Euler X-Y-Z$deg$WORLD$true#Right$CS2$[0 0 0]$CS1$CS1$m$[0 0 0]$Euler X-Y-Z$deg$WORLD$true#Right$CS3$[0 0 0]$CS1$CS1$m$[0 0 0]$Euler X-Y-Z$deg$WORLD$true  CGPos=[0 0 0]  CGRot=[0 0 0]  CS0Pos=[]  CS0Rot=[]  CS1Pos=[0 0 0]  CS1Rot=[0 0 0]  CS2Pos=[0 0 0]  CS2Rot=[0 0 0]  CS3Pos=[0 0 0]  CS3Rot=[0 0 0]  CS4Pos=[]  CS4Rot=[]  CS5Pos=[]  CS5Rot=[]  CS6Pos=[]  CS6Rot=[]  CS7Pos=[]  CS7Rot=[]  CS8Pos=[]  CS8Rot=[]  CS9Pos=[]  CS9Rot=[]  CS10Pos=[]  CS10Rot=[]  CS11Pos=[]  CS11Rot=[]  CS12Pos=[]  CS12Rot=[]  CS13Pos=[]  CS13Rot=[]  CS14Pos=[]  CS14Rot=[]  CS15Pos=[]  CS15Rot=[]  CS16Pos=[]  CS16Rot=[]  CS17Pos=[]  CS17Rot=[]  CS18Pos=[]  CS18Rot=[]  CS19Pos=[]  CS19Rot=[]  CS20Pos=[]  CS20Rot=[]
  Gear Constraint : mblibv1/Constraints &  Drivers/Gear Constraint  Orientation=up  DialogController=MECH.DynMechDlgSource  PhysicalDomain=mechanical  SubClassName=Unknown  LeftPortType=blob  RightPortType=blob  LConnTagsString=__newl0  RConnTagsString=__newr0  DialogClass=GearConstraint  NumSAPorts=0  BaseRadius=1e-2/abs(ig)  BaseRadiusUnits=m  FollowerRadius=1e-2  FollowerRadiusUnits=m
  Housing : mblibv1/Bodies/Body  Orientation=left  DialogController=MECH.DynMechDlgSource  PhysicalDomain=mechanical  SubClassName=Unknown  LeftPortType=workingframe  RightPortType=workingframe  LConnTagsString=CS1  RConnTagsString=CS2|CS3  DialogClass=MechanicalBodyBlock  Mass=0  MassUnits=kg  InertiaUnits=kg*m^2  Inertia=zeros(3,3)  Shape=Cylinder  ShapeDims=[1 1]  ShapeUnits=m  ShapeUse=false  Density=1  DensityUnits=kg/m^3  DensityUse=false  GraphicsMode=1  BodyColor=[0.5 0.5 0.5]  GraphicsObj=[]  AttachedToCS=1  CG=Left$CG$[0 0 0]$CS1$CS1$m$[0 0 0]$Euler X-Y-Z$deg$WORLD$false  WorkingFrames=Left$CS1$[0 0 0]$ADJOINING$ADJOINING$m$[0 0 0]$Euler X-Y-Z$deg$WORLD$true#Right$CS2$[0 0 0]$CS1$CS1$m$[0 0 0]$Euler X-Y-Z$deg$WORLD$true#Right$CS3$Vector$CS1$CS1$m$[0 0 0]$Euler X-Y-Z$deg$WORLD$true  CGPos=[0 0 0]  CGRot=[0 0 0]  CS0Pos=[]  CS0Rot=[]  CS1Pos=[0 0 0]  CS1Rot=[0 0 0]  CS2Pos=[0 0 0]  CS2Rot=[0 0 0]  CS3Pos=Vector  CS3Rot=[0 0 0]  CS4Pos=[]  CS4Rot=[]  CS5Pos=[]  CS5Rot=[]  CS6Pos=[]  CS6Rot=[]  CS7Pos=[]  CS7Rot=[]  CS8Pos=[]  CS8Rot=[]  CS9Pos=[]  CS9Rot=[]  CS10Pos=[]  CS10Rot=[]  CS11Pos=[]  CS11Rot=[]  CS12Pos=[]  CS12Rot=[]  CS13Pos=[]  CS13Rot=[]  CS14Pos=[]  CS14Rot=[]  CS15Pos=[]  CS15Rot=[]  CS16Pos=[]  CS16Rot=[]  CS17Pos=[]  CS17Rot=[]  CS18Pos=[]  CS18Rot=[]  CS19Pos=[]  CS19Rot=[]  CS20Pos=[]  CS20Rot=[]
  Joint Initial Condition1 : mblibv1/Sensors &  Actuators/Joint Initial Condition  Orientation=up  DialogController=MECH.DynMechDlgSource  SystemSampleTime=-1  PhysicalDomain=Mechanical  DialogClass=InitialConditionBlock  Primitive=R1  CoordPosition=q0*ig  Velocity=0.0  AngleUnits=rad  ArcVelocityUnits=deg/s  CoordPositionUnits=m  VelocityUnits=m/s  InitialConditions=P1$false$0$m$rad$0$m/s$rad/s#P2$false$0$m$rad$0$m/s$rad/s#P3$false$0$m$rad$0$m/s$rad/s#R1$true$q0*ig$m$rad$0.0$m/s$deg/s#R2$false$0$m$rad$0$m/s$rad/s#R3$false$0$m$rad$0$m/s$rad/s#S$false$0$m$rad$0$m/s$rad/s  P1PIC=0  P1VIC=0  P2PIC=0  P2VIC=0  P3PIC=0  P3VIC=0  R1PIC=q0*ig  R1VIC=0.0  R2PIC=0  R2VIC=0  R3PIC=0  R3VIC=0  SPIC=0  SVIC=0
  Revolute1 : mblibv1/Joints/Revolute  Tag=Factory generic  Description=Mechanical Blockset  Orientation=left  DialogController=MECH.DynMechDlgSource  PhysicalDomain=mechanical  SubClassName=Unknown  LeftPortType=blob  RightPortType=blob  LConnTagsString=__newl0|SA1|SA2  RConnTagsString=__newr0|SA1  NumSAPorts=3  CutJoint=off  MarkAsCut=off  Primitives=revolute  PrimitiveProps=R1$WORLD$Axis$revolute  DialogClass=JointBlock  R1Axis=Axis
  Revolute2 : mblibv1/Joints/Revolute  Tag=Factory generic  Description=Mechanical Blockset  Orientation=left  DialogController=MECH.DynMechDlgSource  PhysicalDomain=mechanical  SubClassName=Unknown  LeftPortType=blob  RightPortType=blob  LConnTagsString=__newl0|SA1  RConnTagsString=__newr0  NumSAPorts=1  CutJoint=off  MarkAsCut=off  Primitives=revolute  PrimitiveProps=R1$WORLD$Axis$revolute  DialogClass=JointBlock  R1Axis=Axis
  Rotor inertia1 : mblibv1/Bodies/Body  Tag=Factory generic  Description=Mechanical Blockset  Orientation=left  DialogController=MECH.DynMechDlgSource  PhysicalDomain=mechanical  SubClassName=Unknown  LeftPortType=workingframe  RightPortType=workingframe  LConnTagsString=CS1  RConnTagsString=CS2  DialogClass=MechanicalBodyBlock  Mass=0.5  MassUnits=kg  InertiaUnits=kg*m^2  Inertia=diag([Actuator.MotorInertia Actuator.MotorInertia/2 Actuator.MotorInertia/2])  Shape=Cylinder  ShapeDims=[1 1]  ShapeUnits=m  ShapeUse=false  Density=1  DensityUnits=kg/m^3  DensityUse=false  GraphicsMode=1  BodyColor=[0.5 0.5 0.5]  GraphicsObj=[]  AttachedToCS=1  CG=Left$CG$[0 0 0]$CS1$CS1$m$T$3x3 Transform$deg$WORLD$false  WorkingFrames=Left$CS1$[0 0 0]$ADJOINING$ADJOINING$m$[0 0 0]$Euler X-Y-Z$deg$WORLD$true#Right$CS2$[0 0 0]$CS1$CS1$m$[0 0 0]$Euler X-Y-Z$deg$WORLD$true  CGPos=[0 0 0]  CGRot=T  CS0Pos=[]  CS0Rot=[]  CS1Pos=[0 0 0]  CS1Rot=[0 0 0]  CS2Pos=[0 0 0]  CS2Rot=[0 0 0]  CS3Pos=[]  CS3Rot=[]  CS4Pos=[]  CS4Rot=[]  CS5Pos=[]  CS5Rot=[]  CS6Pos=[]  CS6Rot=[]  CS7Pos=[]  CS7Rot=[]  CS8Pos=[]  CS8Rot=[]  CS9Pos=[]  CS9Rot=[]  CS10Pos=[]  CS10Rot=[]  CS11Pos=[]  CS11Rot=[]  CS12Pos=[]  CS12Rot=[]  CS13Pos=[]  CS13Rot=[]  CS14Pos=[]  CS14Rot=[]  CS15Pos=[]  CS15Rot=[]  CS16Pos=[]  CS16Rot=[]  CS17Pos=[]  CS17Rot=[]  CS18Pos=[]  CS18Rot=[]  CS19Pos=[]  CS19Rot=[]  CS20Pos=[]  CS20Rot=[]
  Weld : mblibv1/Joints/Weld  Orientation=left  DialogController=MECH.DynMechDlgSource  PhysicalDomain=mechanical  SubClassName=Unknown  LeftPortType=blob  RightPortType=blob  LConnTagsString=__newl0  RConnTagsString=__newr0  NumSAPorts=0  CutJoint=off  MarkAsCut=off  Primitives=weld  PrimitiveProps=W$INERTIAL$[0 0 0]$weld  DialogClass=JointBlock  WAxis=[0 0 0]
  Weld1 : mblibv1/Joints/Weld  Orientation=left  DialogController=MECH.DynMechDlgSource  PhysicalDomain=mechanical  SubClassName=Unknown  LeftPortType=blob  RightPortType=blob  LConnTagsString=__newl0  RConnTagsString=__newr0  NumSAPorts=0  CutJoint=off  MarkAsCut=off  Primitives=weld  PrimitiveProps=W$INERTIAL$[0 0 0]$weld  DialogClass=JointBlock  WAxis=[0 0 0]
  Base : PMIOPort  Tag=PMCPort  Orientation=left  Port=1  Side=Left
  Follower : PMIOPort  Tag=PMCPort  Port=2  Side=Right
  Sensor : PMIOPort  Orientation=left  Port=3  Side=Left
  Actuator : PMIOPort  Orientation=left  Port=4  Side=Left
  connections:
  Revolute2/LConn2 -- "Continuous angle "/LConn1
  Revolute2/RConn1 -- Gear/LConn1
  Gear/RConn1 -- Weld1/LConn1
  Gear/RConn2 -- Gear Constraint/RConn1
  Rotor inertia1/RConn1 -- Gear Constraint/LConn1
  Weld/RConn1 -- Housing/LConn1
  Revolute2/LConn1 -- Housing/RConn1
  Housing/RConn2 -- Revolute1/LConn1
  Revolute1/RConn1 -- Rotor inertia1/LConn1
  Base/RConn1 -- Weld/LConn1
  Weld1/RConn1 -- Follower/RConn1
  Sensor/RConn1 -- Revolute1/LConn2
  Revolute1/LConn3 -- Actuator/RConn1
  Joint Initial Condition1/RConn1 -- Revolute1/RConn2

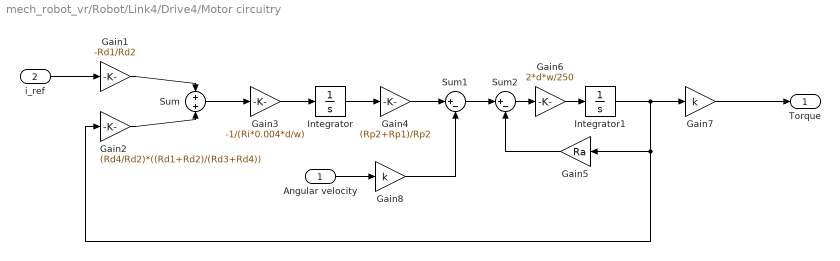
== system mech_robot_vr/Robot/Link4/Drive4/Motor circuitry ==
  Angular velocity : Inport  OutDataType=sfix(16)  OutScaling=2^0
  i_ref : Inport  Port=2  OutDataType=sfix(16)  OutScaling=2^0
  Gain1 : Gain  Gain=-Rd1/Rd2  ParameterDataType=sfix(16)  ParameterScaling=2^0  OutDataType=sfix(16)  OutScaling=2^0  SaturateOnIntegerOverflow=on  OutDataTypeStr=Inherit: Same as input  ParamDataTypeStr=Inherit: Same as input
  Gain2 : Gain  Gain=(Rd4/Rd2)*((Rd1+Rd2)/(Rd3+Rd4))  ParameterDataType=sfix(16)  ParameterScaling=2^0  OutDataType=sfix(16)  OutScaling=2^0  SaturateOnIntegerOverflow=on  OutDataTypeStr=Inherit: Same as input  ParamDataTypeStr=Inherit: Same as input
  Gain3 : Gain  Gain=-1/(Ri*0.004*d/w)  ParameterDataType=sfix(16)  ParameterScaling=2^0  OutDataType=sfix(16)  OutScaling=2^0  SaturateOnIntegerOverflow=on  OutDataTypeStr=Inherit: Same as input  ParamDataTypeStr=Inherit: Same as input
  Gain4 : Gain  Gain=(Rp2+Rp1)/Rp2  ParameterDataType=sfix(16)  ParameterScaling=2^0  OutDataType=sfix(16)  OutScaling=2^0  SaturateOnIntegerOverflow=on  OutDataTypeStr=Inherit: Same as input  ParamDataTypeStr=Inherit: Same as input
  Gain5 : Gain  Orientation=left  Gain=Ra  ParameterDataType=sfix(16)  ParameterScaling=2^0  OutDataType=sfix(16)  OutScaling=2^0  SaturateOnIntegerOverflow=on  OutDataTypeStr=Inherit: Same as input  ParamDataTypeStr=Inherit: Same as input
  Gain6 : Gain  Gain=2*d*w/250  ParameterDataType=sfix(16)  ParameterScaling=2^0  OutDataType=sfix(16)  OutScaling=2^0  SaturateOnIntegerOverflow=on  OutDataTypeStr=Inherit: Same as input  ParamDataTypeStr=Inherit: Same as input
  Gain7 : Gain  Gain=k  ParameterDataType=sfix(16)  ParameterScaling=2^0  OutDataType=sfix(16)  OutScaling=2^0  SaturateOnIntegerOverflow=on  OutDataTypeStr=Inherit: Same as input  ParamDataTypeStr=Inherit: Same as input
  Gain8 : Gain  Gain=k  ParameterDataType=sfix(16)  ParameterScaling=2^0  OutDataType=sfix(16)  OutScaling=2^0  SaturateOnIntegerOverflow=on  OutDataTypeStr=Inherit: Same as input  ParamDataTypeStr=Inherit: Same as input
  Integrator : Integrator  ZeroCross=off
  Integrator1 : Integrator  ZeroCross=off
  Sum : Sum  OutDataType=sfix(16)  OutScaling=2^0  SaturateOnIntegerOverflow=on  InputSameDT=on  OutDataTypeStr=Inherit: Same as first input
  Sum1 : Sum  Inputs=|+-  OutDataType=sfix(16)  OutScaling=2^0  SaturateOnIntegerOverflow=on  InputSameDT=on  OutDataTypeStr=Inherit: Same as first input
  Sum2 : Sum  Inputs=|+-  OutDataType=sfix(16)  OutScaling=2^0  SaturateOnIntegerOverflow=on  InputSameDT=on  OutDataTypeStr=Inherit: Same as first input
  Torque : Outport  OutDataType=sfix(16)  OutScaling=2^0
  wires:
  Angular velocity/1 -> Gain8/1
  Gain8/1 -> Sum1/2
  Gain6/1 -> Integrator1/1
  Sum2/1 -> Gain6/1
  Gain5/1 -> Sum2/2
  Integrator1/1 -> Gain2/1, Gain5/1, Gain7/1
  Sum1/1 -> Sum2/1
  Gain4/1 -> Sum1/1
  Integrator/1 -> Gain4/1
  Gain3/1 -> Integrator/1
  Sum/1 -> Gain3/1
  Gain2/1 -> Sum/2
  Gain1/1 -> Sum/1
  i_ref/1 -> Gain1/1
  Gain7/1 -> Torque/1

== system mech_robot_vr/Robot/Link5/Drive5/Continuous angle ==
  Angular velocity : Inport  Orientation=left  OutDataType=sfix(16)  OutScaling=2^0
  phi : Inport  Orientation=left  Port=2  OutDataType=sfix(16)  OutScaling=2^0
  Continuous Angle : Subsystem  Tag=Factory continuousAngle  Orientation=left  AncestorBlock=mblibv1/Utilities/Continuous Angle  mask{rad=rad, rads=rad/s}
      mask prompts: rad "Angle measured in:"; rads "Rate measured in:"
      mask help: Outputs a continuous, unbounded angle given a discontinuous, bounded angle and the angular velocity. Choose units for the angle and the angular velocity (rate).
      mask Help: web(mech_help('continuousangle'))
      mask StyleString: popup(rad|deg),popup(rad/s|deg/s)
  "phi " : Outport  Orientation=left  OutDataType=sfix(16)  OutScaling=2^0
  "Angular velocity " : Outport  Orientation=left  Port=2  OutDataType=sfix(16)  OutScaling=2^0
  wires:
  phi/1 -> Continuous Angle/1(Angle)
  Angular velocity/1 -> Continuous Angle/2(Rate), "Angular velocity "/1
  Continuous Angle/1(Continuous Angle) -> "phi "/1

== system mech_robot_vr/Robot/Link5/Drive5/Controller ==
  Angular velocity : Inport  OutDataType=sfix(16)  OutScaling=2^0
  phi : Inport  Port=2  OutDataType=sfix(16)  OutScaling=2^0
  w_ref : Inport  Orientation=down  Port=3  OutDataType=sfix(16)  OutScaling=2^0
  phi_ref : Inport  Port=4  OutDataType=sfix(16)  OutScaling=2^0
  Integrator : Integrator  ZeroCross=off
  Lead filter : TransferFcn  Numerator=[340.8*9.95e-3 340.8]  Denominator=[0.56e-3 1]
  Position gain : Gain  Gain=0.3  ParameterDataType=sfix(16)  ParameterScaling=2^0  OutDataType=sfix(16)  OutScaling=2^0  SaturateOnIntegerOverflow=on  OutDataTypeStr=Inherit: Same as input  ParamDataTypeStr=Inherit: Same as input
  Rate controller : TransferFcn  Orientation=up  Numerator=[40e-3 1]  Denominator=[20.2e-3 1]
  Sum : Sum  Inputs=|+-  OutDataType=sfix(16)  OutScaling=2^0  SaturateOnIntegerOverflow=on
  Sum1 : Sum  Inputs=++|  OutDataType=sfix(16)  OutScaling=2^0  SaturateOnIntegerOverflow=on
  Sum2 : Sum  Inputs=|+-  OutDataType=sfix(16)  OutScaling=2^0  SaturateOnIntegerOverflow=on
  Tacho filter : TransferFcn  Numerator=0.03  Denominator="[8.475e-4  1]"
  Taco dynamics : TransferFcn  Numerator=1  Denominator="[1/(2014*2014)   2*0.294/2014  1]"
  Velocity gain : Gain  Orientation=down  Gain=0.03  ParameterDataType=sfix(16)  ParameterScaling=2^0  OutDataType=sfix(16)  OutScaling=2^0  SaturateOnIntegerOverflow=on  OutDataTypeStr=Inherit: Same as input  ParamDataTypeStr=Inherit: Same as input
  i_ref : Outport  OutDataType=sfix(16)  OutScaling=2^0
  wires:
  phi_ref/1 -> Sum/1
  Sum/1 -> Position gain/1
  Position gain/1 -> Sum1/2
  Velocity gain/1 -> Sum1/1
  Sum1/1 -> Sum2/1
  Sum2/1 -> Lead filter/1
  Rate controller/1 -> Sum2/2
  Taco dynamics/1 -> Rate controller/1
  Tacho filter/1 -> Taco dynamics/1
  Angular velocity/1 -> Tacho filter/1
  Lead filter/1 -> Integrator/1
  Integrator/1 -> i_ref/1
  w_ref/1 -> Velocity gain/1
  phi/1 -> Sum/2

== system mech_robot_vr/Robot/Link5/Drive5/Coulomb friction ==
  Motor torque : Inport  Orientation=down  OutDataType=sfix(16)  OutScaling=2^0
  Constant2 : Constant  Orientation=down  Value=Rv0  OutDataType=sfix(16)  OutScaling=2^0
  Constant3 : Constant  Orientation=left  Value=-peak*Rv0  OutDataType=sfix(16)  OutScaling=2^0
  Constant4 : Constant  Orientation=left  Value=peak*Rv0  OutDataType=sfix(16)  OutScaling=2^0
  Gain3 : Gain  Orientation=left  Gain=-1  ParameterDataType=sfix(16)  ParameterScaling=2^0  OutDataType=sfix(16)  OutScaling=2^0  SaturateOnIntegerOverflow=on  OutDataTypeStr=Inherit: Same as input  ParamDataTypeStr=Inherit: Same as input
  Gain4 : Gain  Orientation=left  Gain=Rv1  ParameterDataType=sfix(16)  ParameterScaling=2^0  OutDataType=sfix(16)  OutScaling=2^0  SaturateOnIntegerOverflow=on  OutDataTypeStr=Inherit: Same as input  ParamDataTypeStr=Inherit: Same as input
  Joint Sensor3 : mblibv1/Sensors &  Actuators/Joint Sensor  Description=Mechanical Blockset  Orientation=left  DialogController=MECH.DynMechDlgSource  SystemSampleTime=-1  PhysicalDomain=Mechanical  PortType=blob  Muxed=off  Pose=off  Angle=on  AngleUnits=rad  ArcVelocity=on  ArcVelocityUnits=rad/s  ArcAcceleration=off  ArcAccelerationUnits=deg/s^2  CoordPosition=off  CoordPositionUnits=m  Velocity=off  VelocityUnits=m/s  Acceleration=off  AccelerationUnits=m/s^2  Quaternion=off  QuaternionDT=off  QuaternionDDT=off  QuaternionUnits=off  OutputVector=[ 1 1 1 ]  ActiveIO=on  Width=3  DialogClass=MechanicalSensorBlock  Primitive=R1  Force=off  ForceUnits=N  Torque=on  TorqueUnits=N-m  ReferenceFrame=Absolute (INERTIAL)  ReactionSensedSide=Base  ReactionReferenceFrame=Absolute (World)  ReactionForce=off  ReactionForceUnits=N  ReactionMoment=off  ReactionMomentUnits=N-m
  Joint Stiction Actuator : mblibv1/Sensors &  Actuators/Joint Stiction Actuator  Description=Mechanical Blockset  Orientation=left  DialogController=MECH.DynMechDlgSource  SystemSampleTime=-1  PhysicalDomain=Mechanical  PortType=blob  ActuationStyle=Force  AngleUnits=deg  ArcVelocityUnits=deg/s  ArcAccelerationUnits=deg/s^2  CoordPositionUnits=m  VelocityUnits=m/s  AccelerationUnits=m/s^2  ForceUnits=N  TorqueUnits=N-m  ActiveIO=on  Width=5  DialogClass=EventActuatorBlock  Primitive=R1  FrictionalForceUnits=N  ExternalForceUnits=N  FrictionalTorqueUnits=N-m  ExternalTorqueUnits=N-m  LockingTolerance=1e-3
  Product : Product  Orientation=left  OutDataType=sfix(16)  OutScaling=2^0  SaturateOnIntegerOverflow=on  InputSameDT=on  OutDataTypeStr=Inherit: Same as first input
  Sign : Signum  Orientation=left
  Sum : Sum  Orientation=left  Inputs=++|  OutDataType=sfix(16)  OutScaling=2^0  SaturateOnIntegerOverflow=on  InputSameDT=on  OutDataTypeStr=Inherit: Same as first input
  Sum1 : Sum  Orientation=left  Inputs=|+-  OutDataType=sfix(16)  OutScaling=2^0  SaturateOnIntegerOverflow=on  InputSameDT=on  OutDataTypeStr=Inherit: Same as first input
  Sensor : PMIOPort  Orientation=left  Port=1  Side=Right
  Actuator : PMIOPort  Port=2  Side=Right
  phi : Outport  OutDataType=sfix(16)  OutScaling=2^0
  Angular velocity : Outport  Port=2  OutDataType=sfix(16)  OutScaling=2^0
  wires:
  Sum1/1 -> Joint Stiction Actuator/4
  Constant3/1 -> Joint Stiction Actuator/3
  Gain3/1 -> Product/2
  Constant2/1 -> Sum/1
  Gain4/1 -> Sum/2
  Constant4/1 -> Joint Stiction Actuator/5
  Sum/1 -> Product/1
  Sign/1 -> Gain3/1
  Product/1 -> Joint Stiction Actuator/2
  Motor torque/1 -> Joint Stiction Actuator/1, Sum1/2
  Joint Sensor3/2 -> Sign/1, Gain4/1, Angular velocity/1
  Joint Sensor3/3 -> Sum1/1
  Joint Sensor3/1 -> phi/1
  connections:
  Sensor/RConn1 -- Joint Sensor3/LConn1
  Actuator/RConn1 -- Joint Stiction Actuator/RConn1
